simulink model "LAB5"  (R2016b)
settings: Solver=ode3  StartTime=0.0  StopTime=10.001  FixedStep=2e-6  RelTol=1e-5  EnableMultiTasking=on
libraries: commfilt2 x1, commchan3 x1, commsink2 x1, commrandsrc2 x1
settings Model: Creator=Dennis Silage  LastModifiedBy=avile
settings DataIOCC: LimitDataPoints=on  SaveFormat=Array  SignalLoggingSaveFormat=ModelDataLogs
settings OptimizationCC: ExpressionDepthLimit=2147483647  InitFltsAndDblsToZero=on  LifeSpan=inf
settings DebuggingCC: UnderspecifiedInitializationDetection=Classic  MergeDetectMultiDrivingBlocksExec=none  FcnCallInpInsideContextMsg=warning  StateNameClashWarn=warning  SFUnexpectedBacktrackingDiag=warning  SFNoUnconditionalDefaultTransitionDiag=warning  SFExecutionAtInitializationDiag=none
settings HardwareCC: ProdBitPerPointer=32  ProdBitPerSizeT=32  ProdBitPerPtrDiffT=32  ProdLargestAtomicFloat=None  ProdIntDivRoundTo=Undefined  ProdEndianess=Unspecified  ProdWordSize=32  ProdHWDeviceType=32-bit Generic
settings ModelReferenceCC: PropagateSignalLabelsOutOfModel=off
settings GRTTargetCC: TargetLangStandard=C89/C90 (ANSI)  GeneratePreprocessorConditionals=Disable all  CombineOutputUpdateFcns=off  GRTInterface=on
settings ConfigComp: CovMetricSettings=dw  CovHtmlReporting=on  CovSaveCumulativeToWorkspaceVar=on  CovSaveSingleToWorkspaceVar=on  CovExternalEMLEnable=off  CovSFcnEnable=off

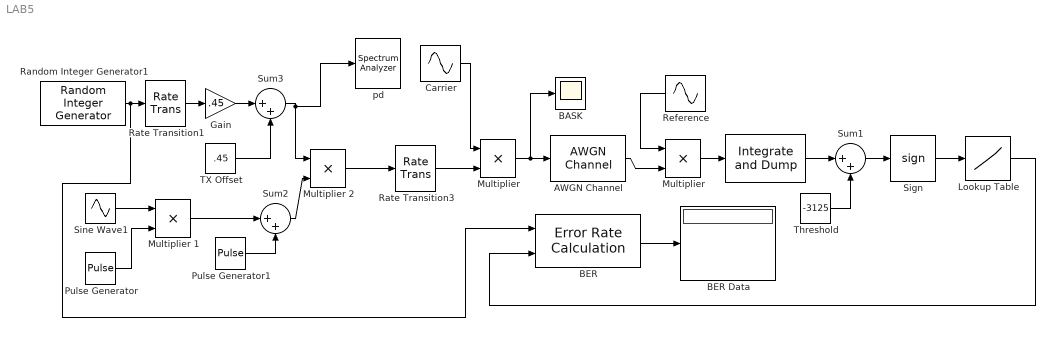
== system LAB5 ==
  " " : commfilt2/Integrate and Dump  obssamples=500  offsetsamples=0  nodump=off  roundingMode=Floor  overflowMode=off  outputDataTypeStr=Inherit: Same as accumulator  outputLastDataTypeStr=Inherit: Same as accumulator
  AWGN Channel : commchan3/AWGN Channel  InputProcessing=Inherited (this choice will be removed - see release notes)  seed=randseed  noiseMode="Signal to noise ratio  (Eb/No)"  EbNodB=12  EsNodB=10  SNRdB=12  bitsPerSym=1  Ps=12.5  Tsym=1e-3  variance=0
  BASK : Scope
  BER : commsink2/Error Rate Calculation  N=2  st_delay=0  cp_mode=Entire frame  subframe=[]  PMode=Port  WsName=ErrorVec  RsMode2=off  stop=off  numErr=100  maxBits=1e6
  BER Data : Display
  Carrier : Sin  Amplitude=5  Frequency=40000*pi  SampleTime=2e-6
  Gain : Gain  Gain=.45
  Lookup Table : Lookup_n-D  NumberOfTableDimensions=1  BreakpointsForDimension1=[-1, 0, 1]  BreakpointsForDimension3=[5, 7]  Table=[0, 0, 1]  InternalRulePriority=Speed  RndMeth=Simplest  InputSameDT=on
  Multiplier : Product  RndMeth=Zero
  "Multiplier " : Product  RndMeth=Zero
  Multiplier 1 : Product  RndMeth=Zero
  Multiplier 2 : Product  RndMeth=Zero
  "Pulse Generator " : DiscretePulseGenerator  PulseType=Time based  Period=.001  PulseWidth=25
  Pulse Generator1 : DiscretePulseGenerator  PulseType=Time based  Period=.001  PulseWidth=75  PhaseDelay=250e-6
  Random Integer Generator1 : commrandsrc2/Random Integer Generator  mul=2  seed=randseed  Ts=1e-3  frameBased=off  sampPerFrame=50  orient=on  outDataType=double
  Rate Transition1 : RateTransition  OutPortSampleTime=2e-6
  Rate Transition3 : RateTransition  OutPortSampleTime=2e-6
  Reference : Sin  Amplitude=5  Frequency=40000*pi  Samples=200  SampleTime=2e-6
  Sign : Signum
  Sine Wave1 : Sin  Frequency=1000*2*pi  SampleTime=0
  Sum1 : Sum  Inputs=|++
  Sum2 : Sum  Inputs=|++
  Sum3 : Sum  Inputs=|++
  TX Offset : Constant  Value=.45
  Threshold : Constant  Value=-3125
  pd : SpectrumAnalyzer
  wires:
  Sign/1 -> Lookup Table/1
  BER/1 -> BER Data/1
  Multiplier/1 -> " "/1
  AWGN Channel/1 -> Multiplier/2
  Threshold/1 -> Sum1/2
  Sum1/1 -> Sign/1
  " "/1 -> Sum1/1
  Reference/1 -> Multiplier/1
  Carrier/1 -> "Multiplier "/1
  Lookup Table/1 -> BER/2
  Sine Wave1/1 -> Multiplier 1/1
  Sum2/1 -> Multiplier 2/2
  Multiplier 1/1 -> Sum2/1
  Pulse Generator1/1 -> Sum2/2
  "Pulse Generator "/1 -> Multiplier 1/2
  Gain/1 -> Sum3/1
  TX Offset/1 -> Sum3/2
  Sum3/1 -> pd/1, Multiplier 2/1
  Rate Transition1/1 -> Gain/1
  "Multiplier "/1 -> AWGN Channel/1, BASK/1
  Multiplier 2/1 -> Rate Transition3/1
  Rate Transition3/1 -> "Multiplier "/2
  Random Integer Generator1/1 -> BER/1, Rate Transition1/1
